simulink model "dc_motor"  (R2021a)
settings: Solver=VariableStepAuto  StartTime=0.0  StopTime=20  FixedStep=Sim.samplingTime  RelTol=1e-3  EnableMultiTasking=on
undefined symbols (not defined in the file): Sim
libraries: adrc_toolbox_library x1, arduinomotorcarrierlib x1, mkrmotorcarrierlib x1
settings Model: SimulationMode=external  SILPILModeSetting=veronly  ExtModeTrigDuration=2  Creator=Krzysztof  LastModifiedBy=krzys
settings SolverCC: AlgebraicLoopSolver=TrustRegion
settings DataIOCC: SaveFormat=StructureWithTime
settings OptimizationCC: EnhancedBackFolding=on  PassReuseOutputArgsThreshold=0  MaxStackSize=64  OptimizeBlockOrder=speed  DifferentSizesBufferReuse=on  OptimizationCustomize=off
settings DebuggingCC: ParameterTunabilityLossMsg=error  SFMachineParentedDataDiag=warning
settings HardwareCC: ProdBitPerPointer=32  ProdBitPerSizeT=32  ProdBitPerPtrDiffT=32  ProdLargestAtomicInteger=Long  ProdLargestAtomicFloat=Double  ProdWordSize=32  ProdLongLongMode=on  ProdHWDeviceType=ARM Compatible->ARM Cortex  UseEmbeddedCoderFeatures=off  UseSimulinkCoderFeatures=off
settings SFSimCC: MATLABDynamicMemAlloc=off
settings RTWCC: SystemTargetFile=ert.tlc  HardwareBoard=Arduino MKR WiFi 1010  TemplateMakefile=ert_default_tmf  Toolchain=Arduino ARM  BuildConfiguration=Faster Runs
settings CodeAppCC: ForceParamTrailComments=on  OperatorAnnotations=on  MangleLength=10
settings ERTTargetCC: ERTCustomFileBanners=off  SupportContinuousTime=on  SupportNonInlinedSFcns=on  RemoveResetFunc=off  SupportVariableSizeSignals=on  ModelStepFunctionPrototypeControlCompliant=off  ExtModeStaticAllocSize=8192

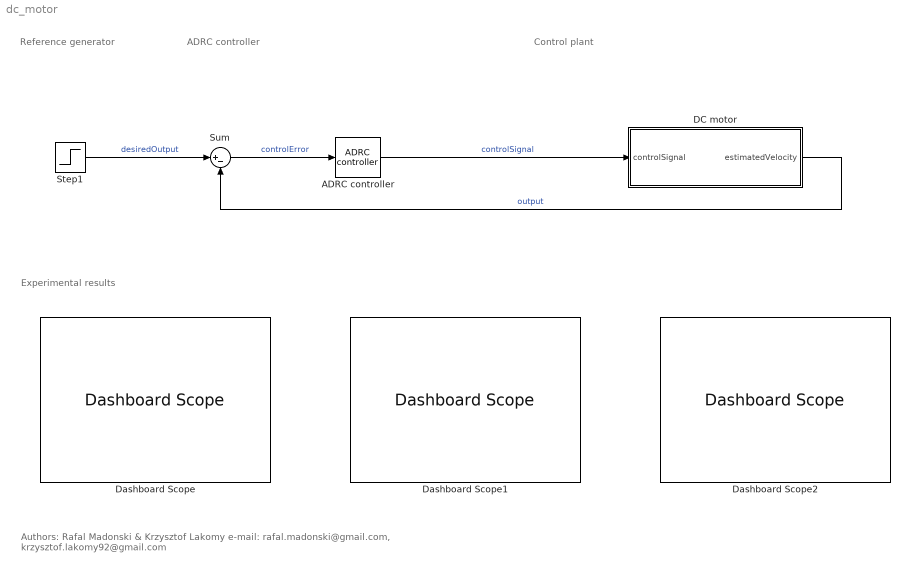
== system dc_motor ==
  note: ADRC controller
  note: Control plant
  note: Reference
      | generator
  note: Experimental results
  note: Authors:  Rafal Madonski & Krzysztof Lakomy
      | e-mail: rafal.madonski@gmail.com, krzysztof.lakomy92@gmail.com
  ADRC controller : adrc_toolbox_library/ADRC controller  dynamicsOrder=1  controllerBandwidth=5  controllerBandwidthSource=Internal  observerBandwidth=50  observerBandwidthSource=Internal  inputGainParameter=800  inputGainSource=Internal  saturationEnabled=on  UpperLimit=100  LowerLimit=-100  antiPeakingEnabled=off  antiPeakingTime=0.2
      link override State feedback robust controller/Saturation: VariantControlMode=label  LabelModeActiveChoice=saturation_off
      settings: SourceProductName=ADRC toolbox
  DC motor : Subsystem
  Dashboard Scope : DashboardScope
  Dashboard Scope1 : DashboardScope
  Dashboard Scope2 : DashboardScope  Ymin=-0.1  Ymax=0.1
  Step1 : Step  Time=3  After=3500  SampleTime=0
  Sum : Sum  Inputs=|+-
  wires:
  Sum/1 -> ADRC controller/1  "controlError"
  Step1/1 -> Sum/1  "desiredOutput"
  DC motor/1(estimatedVelocity) -> Sum/2  "output"
  ADRC controller/1 -> DC motor/1(controlSignal)  "controlSignal"

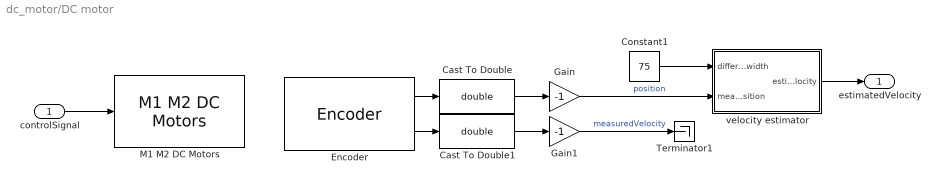
== system dc_motor/DC motor ==
  controlSignal : Inport
  Cast To Double : DataTypeConversion  OutDataTypeStr=double
  Cast To Double1 : DataTypeConversion  OutDataTypeStr=double
  Constant1 : Constant  Value=75  OutDataTypeStr=double
  Encoder : arduinomotorcarrierlib/Encoder  SlaveAddress=uint8( hex2dec( '66' ) )  blockPlatform=ARDUINO  Encoder=1  ShowSpeed=on  ResetOption=on  SampleTime=0.01
      settings: SourceProductBaseCode=ARDUINO
  Gain : Gain  Gain=-1  OutDataTypeStr=double
  Gain1 : Gain  Gain=-1  ParamDataTypeStr=double
  M1 M2 DC Motors : mkrmotorcarrierlib/M1 M2 DC Motors  SlaveAddress=uint8( hex2dec( '66' ) )  blockPlatform=ARDUINO  MotorNumber=M1  MotorCarrierPWMFreq=100
      settings: SourceProductBaseCode=ARDUINO
  Terminator1 : Terminator
  velocity estimator : Subsystem
  estimatedVelocity : Outport
  wires:
  Cast To Double/1 -> Gain/1
  Gain/1 -> velocity estimator/2(measuredPosition)  "position"
  Encoder/2 -> Cast To Double1/1
  velocity estimator/1(estimatedVelocity) -> estimatedVelocity/1
  Cast To Double1/1 -> Gain1/1
  Constant1/1 -> velocity estimator/1(differentiatorBandwidth)
  Gain1/1 -> Terminator1/1  "measuredVelocity"
  Encoder/1 -> Cast To Double/1
  controlSignal/1 -> M1 M2 DC Motors/1

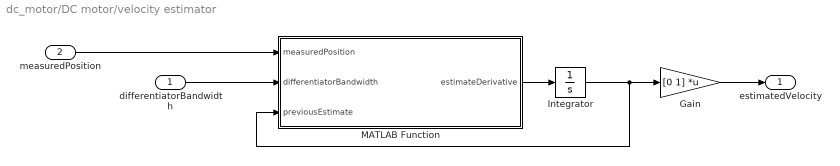
== system dc_motor/DC motor/velocity estimator ==
  differentiatorBandwidth : Inport
  measuredPosition : Inport  Port=2
  Gain : Gain  Gain=[0 1]  Multiplication=Matrix(K*u)
  Integrator : Integrator  InitialCondition=[0;0]
  MATLAB Function : MATLAB Function  TreatAsAtomicUnit=on  SystemSampleTime=Sim.samplingTime
  estimatedVelocity : Outport
  wires:
  MATLAB Function/1(estimateDerivative) -> Integrator/1
  Integrator/1 -> Gain/1, MATLAB Function/3(previousEstimate)
  measuredPosition/1 -> MATLAB Function/1(measuredPosition)
  differentiatorBandwidth/1 -> MATLAB Function/2(differentiatorBandwidth)
  Gain/1 -> estimatedVelocity/1

== matlab function dc_motor/DC motor/velocity estimator/MATLAB Function ==
  data: measuredPosition input; estimateDerivative output; differentiatorBandwidth input; previousEstimate input
function estimateDerivative = fcn(measuredPosition, differentiatorBandwidth, previousEstimate)
    stateMatrix = [0 1; 0 0];
    gainVector = [2 * differentiatorBandwidth; differentiatorBandwidth ^ 2];

    estimateDerivative = stateMatrix * previousEstimate + gainVector * (measuredPosition - previousEstimate(1));
end
